simulink model "TestRpi"  (R2024a)
settings: Solver=FixedStepAuto  StartTime=0.0  StopTime=10000  RelTol=1e-3  EnableMultiTasking=on
libraries: raspberrypiBasiclib x2
settings Model: PacingRate=112  ExtModeTrigDuration=2  Creator=user  LastModifiedBy=user
settings SolverCC: PositivePriorityOrder=on
settings OptimizationCC: EnhancedBackFolding=on  PassReuseOutputArgsAs=Individual arguments  ZeroExternalMemoryAtStartup=off  ZeroInternalMemoryAtStartup=off  MaxStackSize=64  OptimizeBlockOrder=speed  DifferentSizesBufferReuse=on  OptimizationCustomize=off  EfficientTunableParamExpr=on
settings DebuggingCC: ParameterTunabilityLossMsg=error
settings HardwareCC: ProdBitPerLong=64  ProdLargestAtomicInteger=LongLong  ProdLargestAtomicFloat=Double  ProdLongLongMode=on  ProdHWDeviceType=ARM Compatible->ARM 64-bit (LP64)
settings RTWCC: Description=Embedded Coder  SystemTargetFile=ert.tlc  HardwareBoard=Raspberry Pi (64bit)  TLCOptions="-aInlineSetEventsForThisBaseRateFcn=TLC_FALSE -aSuppressMultiTaskScheduler=TLC_FALSE  -aRateBasedStepFcn=0"  TemplateMakefile=ert_default_tmf  Toolchain=GNU GCC Embedded Linux  BuildConfiguration=Faster Runs
settings CodeAppCC: ForceParamTrailComments=on  IgnoreCustomStorageClasses=off  OperatorAnnotations=on  SimulinkDataObjDesc=on  SFDataObjDesc=on  InsertBlockDesc=on
settings ERTTargetCC: SupportContinuousTime=on  SupportVariableSizeSignals=on

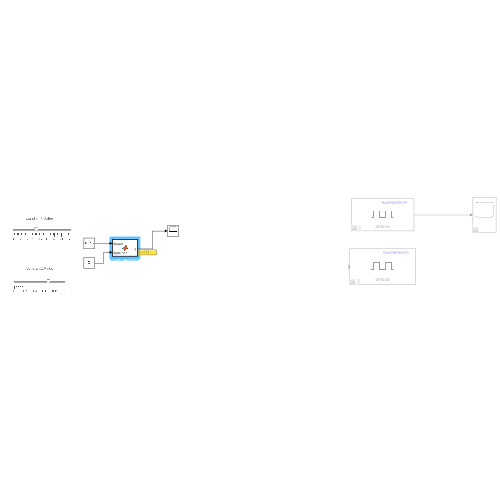
[thumbnail: Simulink's stored preview of the top-level diagram]
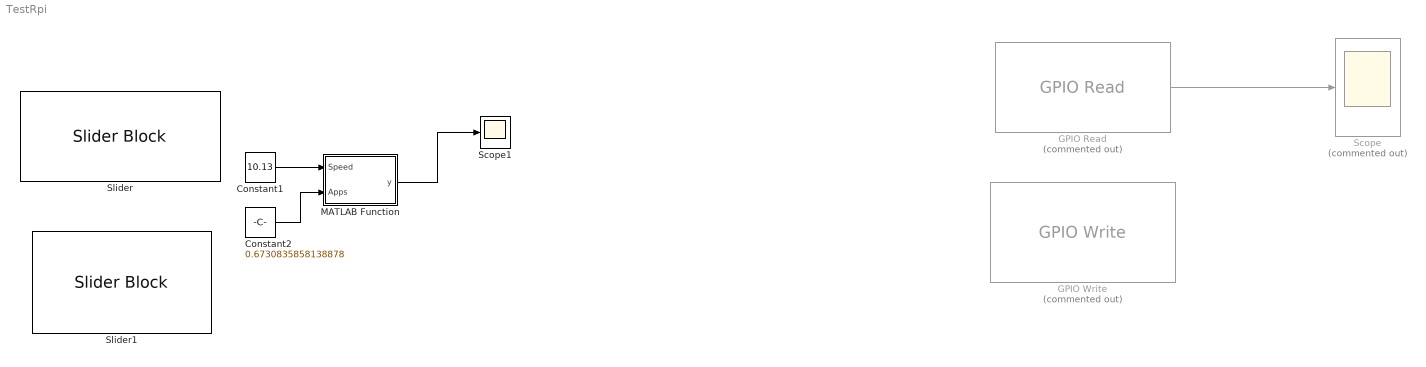
== system TestRpi ==
  Constant1 : Constant  Value=10.13
  Constant2 : Constant  Value=0.6730835858138878
  GPIO Read : raspberrypiBasiclib/GPIO Read  Commented=on  board=Pi Zero 2 W  gpio=19  internalResistor=Off  sampleTime=1  direction=Input  blockPlatform=Raspberry Pi
  GPIO Write : raspberrypiBasiclib/GPIO Write  Commented=on  board=Pi Zero 2 W  gpio=26  direction=Output  blockPlatform=Raspberry Pi
  MATLAB Function : MATLAB Function  TreatAsAtomicUnit=on
  Scope : Scope  Commented=on
  Scope1 : Scope
  Slider : SliderBlock  ScaleMax=25
  Slider1 : SliderBlock  ScaleMax=1
  wires:
  GPIO Read/1 -> Scope/1
  Constant1/1 -> MATLAB Function/1(Speed)
  MATLAB Function/1(y) -> Scope1/1
  Constant2/1 -> MATLAB Function/2(Apps)

== matlab function TestRpi/MATLAB Function ==
  data: Speed input; y output; Apps input
function y= fcn(Speed, Apps)
persistent prev_state;  % Retains value between function calls
    if isempty(prev_state)
        prev_state = 0;  % Initialize only once
    end
if(Speed>10.14) || (Speed<10.12)
    y = Apps;
    prev_state = Apps;
else
    if(Apps >= prev_state-0.1) && (Apps<=prev_state+0.3)
        y = prev_state;
    else
        y = Apps;
        prev_state = Apps;
    end
end
